simulink model "DrivetrainHevMm"  (R2020a)
settings: Solver=VariableStepAuto  StartTime=0.0  StopTime=inf  RelTol=1e-3  EnableMultiTasking=on
model workspace (MAT data in the model file):
  DiffRatio = 3.421
  EngDriveRatio = 0.813008130081
  Jengine = 0.22
  MotGbRatio = 2.45
  NF = Simulink.Parameter
  NF.Value = 2
  NF.DataType = 'auto'
  NF.Dimensions = [1 1]
  NR = Simulink.Parameter
  NR.Value = 2
  NR.DataType = 'auto'
  NR.Dimensions = [1 1]
  RWheel = 0.3
  b_axle = Simulink.Parameter
  b_axle.Value = 10
  b_axle.DataType = 'auto'
  b_axle.Dimensions = [1 1]
  b_driveshaft = Simulink.Parameter
  b_driveshaft.Value = 10
  b_driveshaft.DataType = 'auto'
  b_driveshaft.Dimensions = [1 1]
  k_axle = Simulink.Parameter
  k_axle.Value = 5000
  k_axle.DataType = 'auto'
  k_axle.Dimensions = [1 1]
  k_driveshaft = Simulink.Parameter
  k_driveshaft.Value = 1000
  k_driveshaft.DataType = 'auto'
  k_driveshaft.Dimensions = [1 1]
  wc_shaft = Simulink.Parameter
  wc_shaft.Value = 1000
  wc_shaft.DataType = 'auto'
  wc_shaft.Dimensions = [1 1]
libraries: autolibpowerinfoutils x8, autolibsharedcoupling x7, autolibshareddiff x4, autolibshared x3, autolibtransamt x1
(part 1 of 3)
settings Model: ModifiedByFormat=The MathWorks, Inc.  SimulationMode=accelerator  PauseTimes=10  Creator=The MathWorks, Inc.  LastModifiedBy=The MathWorks, Inc.
settings SolverCC: DecoupledContinuousIntegration=on
settings DataIOCC: DSMLogging=off  ReturnWorkspaceOutputs=off
settings DebuggingCC: MergeDetectMultiDrivingBlocksExec=none  ArithmeticOperatorsInVariantConditions=warning
settings ModelReferenceCC: PropagateSignalLabelsOutOfModel=off
settings SFSimCC: SimUseLocalCustomCode=off  CustomCodeUndefinedFunction=UseInterfaceOnly
settings RTWCC: RTWUseLocalCustomCode=off
settings CodeAppCC: StateflowObjectComments=on
settings GRTTargetCC: TargetLangStandard=C89/C90 (ANSI)
settings ConfigComp: CovMetricSettings=dsw  CovHtmlReporting=on  CovSaveCumulativeToWorkspaceVar=on  CovSaveSingleToWorkspaceVar=on  CovShowResultsExplorer=off  CovExternalEMLEnable=off
settings SimscapeCC: SimscapeNormalizeSystem=off  SimscapeNominalValues={1, 'bar'; 1, 'cm^3/s'; 1, 'bar*kg/s'; 1, 'kJ/kg'; 1, 'kW'; }

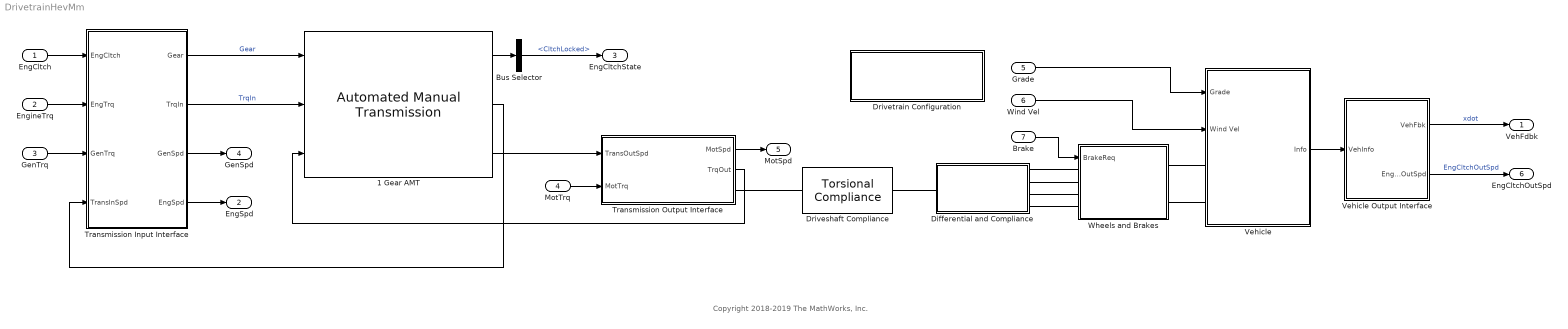
== system DrivetrainHevMm ==
  note: Copyright 2018-2019 The MathWorks, Inc.
  EngCltch : Inport  OutDataTypeStr=boolean
  EngineTrq : Inport  Port=2
  GenTrq : Inport  Port=3
  MotTrq : Inport  Port=4
  Grade : Inport  Port=5
  Wind Vel : Inport  Port=6
  Brake : Inport  Port=7
  1 Gear AMT : autolibtransamt/Automated Manual Transmission  VariantControl=0  cntrlType=Ideal integrated controller  TransEffModelPopup=Gear only  Jin=Jengine  bin=.0011  omegain_o=0  G=[0, 1]  Trq_bpts=[25, 50, 75, 100, 150, 200, 250]  omega_bpts=[52.4 78.5 105 131 157 183 209 262 314 419 524]  Temp_bpts=[313 358]  N=[EngDriveRatio EngDriveRatio]  Jout=[0.03 0.03]  bout=[.001 .001]  eta=[0.95, 0.95]  eta_tbl=reshape([0.53 0.71 0.77 0.79 0.82 0.82 0.82 0.5 0.7 0.77 0.79 0.82 0.82 0.82 0.54 0.72 0.78 0.81 0.83 0.82 0.82 0.56 0.73 0.79 0.81 0.84 0.82 0.82 0.58 0.74 0.79 0.82 0.84 0.82 0.82 0.57 0.74 0.79 0.82 0.84 0.82 0.82 0.58 0.74 0.79 0.82 0.84 0.82 0.82 0.58 0.74 0.79 0.82 0.84 0.82 0.82 0.57 0.74 0.8 0.82 0.85 0.82 0.82 0.55 0.73 0.78 0.81 0.84 0.82 0.82 0.51 0.71 0.77 0.81 0.84 0.82 0.82 0.53 0.71 0.77 0.79 0.82 0.82 0.82 0.5 0.7 0.77 0.79 0.82 0.82 0.82 0.54 0.72 0.78 0.81 0.83 0.82 0.82 0.56 0.73 0.79 0.81 0.84 0.82 0.82 0.58 0.74 0.79 0.82 0.84 0.82 0.82 0.57 0.74 0.79 0.82 0.84 0.82 0.82 0.58 0.74 0.79 0.82 0.84 0.82 0.82 0.58 0.74 0.79 0.82 0.84 0.82 0.82 0.57 0.74 0.8 0.82 0.85 0.82 0.82 0.55 0.73 0.78 0.81 0.84 0.82 0.82 0.51 0.71 0.77 0.81 0.84 0.82 0.82 0.53 0.71 0.77 0.79 0.82 0.82 0.82 0.5 0.7 0.77 0.79 0.82 0.82 0.82 0.54 0.72 0.78 0.81 0.83 0.82 0.82 0.56 0.73 0.79 0.81 0.84 0.82 0.82 0.58 0.74 0.79 0.82 0.84 0.82 0.82 0.57 0.74 0.79 0.82 0.84 0.82 0.82 0.58 0.74 0.79 0.82 0.84 0.82 0.82 0.58 0.74 0.79 0.82 0.84 0.82 0.82 0.57 0.74 0.8 0.82 0.85 0.82 0.82 0.55 0.73 0.78 0.81 0.84 0.82 0.82 0.51 0.71 0.77 0.81 0.84 0.82 0.82 0.7 0.79 0.82 0.83 0.84 0.84 0.84 0.63 0.76 0.8 0.82 0.83 0.84 0.84 0.58 0.74 0.79 0.81 0.83 0.84 0.84 0.58 0.74 0.79 0.81 0.83 0.84 0.84 0.58 0.74 0.79 0.81 0.84 0.84 0.84 0.57 0.73 0.78 0.81 0.84 0.85 0.84 0.57 0.73 0.79 0.81 0.84 0.85 0.84 0.56 0.73 0.78 0.81 0.83 0.85 0.84 0.55 0.73 0.78 0.81 0.84 0.85 0.84 0.52 0.71 0.77 0.8 0.83 0.85 0.84 0.48 0.69 0.76 0.79 0.83 0.84 0.84 0.64 0.76 0.8 0.81 0.83 0.84 0.84 0.56 0.73 0.78 0.8 0.83 0.84 0.84 0.54 0.71 0.77 0.8 0.82 0.84 0.84 0.53 0.71 0.77 0.8 0.83 0.84 0.84 0.51 0.71 0.77 0.8 0.83 0.84 0.85 0.52 0.7 0.77 0.8 0.83 0.84 0.85 0.51 0.71 0.76 0.79 0.83 0.84 0.85 0.5 0.69 0.76 0.79 0.82 0.84 0.85 0.45 0.68 0.75 0.78 0.82 0.84 0.85 0.43 0.67 0.74 0.78 0.81 0.83 0.84 0.38 0.63 0.71 0.75 0.8 0.82 0.83 0.65 0.79 0.84 0.85 0.88 0.89 0.89 0.56 0.75 0.81 0.83 0.86 0.88 0.89 0.52 0.72 0.79 0.83 0.86 0.88 0.88 0.51 0.72 0.79 0.83 0.86 0.88 0.89 0.49 0.71 0.78 0.82 0.86 0.88 0.89 0.47 0.7 0.78 0.82 0.86 0.87 0.88 0.45 0.69 0.77 0.81 0.85 0.87 0.88 0.4 0.67 0.75 0.8 0.84 0.86 0.88 0.3 0.64 0.73 0.78 0.83 0.86 0.87 0.17 0.55 0.67 0.73 0.8 0.83 0.85 0.089 0.45 0.61 0.69 0.77 0.81 0.83 0.61 0.75 0.82 0.84 0.87 0.87 0.88 0.54 0.73 0.8 0.82 0.86 0.87 0.88 0.51 0.71 0.79 0.82 0.86 0.87 0.88 0.52 0.72 0.79 0.82 0.86 0.87 0.89 0.52 0.72 0.8 0.83 0.86 0.88 0.89 0.53 0.72 0.79 0.82 0.86 0.87 0.89 0.5 0.7 0.78 0.82 0.86 0.88 0.88 0.46 0.69 0.77 0.81 0.85 0.87 0.88 0.4 0.67 0.75 0.8 0.83 0.86 0.88 0.33 0.64 0.73 0.78 0.83 0.85 0.87 0.33 0.64 0.73 0.78 0.83 0.85 0.87 0.78 0.85 0.87 0.88 0.89 0.89 0.89 0.73 0.83 0.86 0.88 0.89 0.89 0.89 0.72 0.83 0.86 0.88 0.89 0.89 0.89 0.72 0.83 0.87 0.89 0.9 0.89 0.89 0.72 0.83 0.87 0.88 0.9 0.89 0.89 0.71 0.83 0.87 0.88 0.9 0.89 0.89 0.71 0.83 0.86 0.88 0.9 0.89 0.89 0.7 0.82 0.86 0.88 0.9 0.89 0.89 0.69 0.82 0.86 0.88 0.9 0.89 0.89 0.67 0.81 0.86 0.88 0.9 0.89 0.89 0.63 0.79 0.85 0.87 0.89 0.89 0.89 0.78 0.85 0.87 0.88 0.89 0.89 0.89 0.73 0.83 0.86 0.88 0.89 0.89 0.89 0.72 0.83 0.86 0.88 0.89 0.89 0.89 0.72 0.83 0.87 0.89 0.9 0.89 0.89 0.72 0.83 0.87 0.88 0.9 0.89 0.89 0.71 0.83 0.87 0.88 0.9 0.89 0.89 0.71 0.83 0.86 0.88 0.9 0.89 0.89 0.7 0.82 0.86 0.88 0.9 0.89 0.89 0.69 0.82 0.86 0.88 0.9 0.89 0.89 0.67 0.81 0.86 0.88 0.9 0.89 0.89 0.63 0.79 0.85 0.87 0.89 0.89 0.89 0.78 0.85 0.87 0.88 0.89 0.89 0.89 0.73 0.83 0.86 0.88 0.89 0.89 0.89 0.72 0.83 0.86 0.88 0.89 0.89 0.89 0.72 0.83 0.87 0.89 0.9 0.89 0.89 0.72 0.83 0.87 0.88 0.9 0.89 0.89 0.71 0.83 0.87 0.88 0.9 0.89 0.89 0.71 0.83 0.86 0.88 0.9 0.89 0.89 0.7 0.82 0.86 0.88 0.9 0.89 0.89 0.69 0.82 0.86 0.88 0.9 0.89 0.89 0.67 0.81 0.86 0.88 0.9 0.89 0.89 0.63 0.79 0.85 0.87 0.89 0.89 0.89 0.82 0.87 0.88 0.89 0.89 0.89 0.89 0.81 0.87 0.89 0.89 0.9 0.9 0.89 0.76 0.85 0.87 0.89 0.9 0.89 0.89 0.72 0.83 0.86 0.88 0.89 0.89 0.89 0.72 0.83 0.86 0.88 0.89 0.9 0.89 0.71 0.82 0.86 0.88 0.89 0.9 ...(+1314 chars))  omegaout_o=0  G_o=0  tauc=.02  ts=0.02  tc=.5  R=.2  K_c=5e3  mus=0.35  muk=0.3  ClutchLocked=off  SynchLocked=off  maxAbsSpd=5e3
      settings: SourceProductBaseCode=PW
  Bus Selector : BusSelector  OutputSignals=Cltch.CltchLocked
  Differential and Compliance : Subsystem  Variant=on  VariantControlMode=Label  LabelModeActiveChoice=0
  Driveshaft Compliance : autolibsharedcoupling/Torsional Compliance  port_config=Two-way connection  extInfo=off  k=k_driveshaft  b=b_driveshaft  theta_o=0  domega_o=0  omega_c=wc_shaft  blkID=0  aMode=1
      settings: SourceProductBaseCode=PW,MT,VE,VP
  Drivetrain Configuration : Subsystem  mask(Drivetrain Configuration){drivetrainMode=Front Wheel Drive}
      mask prompts: drivetrainMode "Drivetrain Mode"
      mask help: Use this block to configure the dirvetrain mode.
      settings: AttributesFormatString=Active Mode: %<drivetrainMode>
      mask TypeOptions drivetrainMode: Front Wheel Drive | Rear Wheel Drive | All Wheel Drive
      mask Callback drivetrainMode:
      | switch get_param(gcb,'drivetrainMode')
      |     case 'Front Wheel Drive'
      |         set_param([bdroot '/Differential and Compliance'],'OverrideUsingVariant','0')
      |     case 'Rear Wheel Drive'
      |         set_param([bdroot '/Differential and Compliance'],'OverrideUsingVariant','1')
      |     case 'All Wheel Drive'
      |         set_param([bdroot '/Differential and Compliance'],'OverrideUsingVariant','2')
      |     otherwise
      |         set_param([bdroot '/Differential and Compliance'],'OverrideUsingVariant','0')
      | end
      mask Display: disp('Double click to configure drivetrain')
  Transmission Input Interface : Subsystem
  Transmission Output Interface : Subsystem
  Vehicle : Subsystem
  Vehicle Output Interface : Subsystem
  Wheels and Brakes : Subsystem  VariantControl=0
  VehFdbk : Outport  VectorParamsAs1DForOutWhenUnconnected=off
  EngSpd : Outport  Port=2  VectorParamsAs1DForOutWhenUnconnected=off  BusOutputAsStruct=on
  EngCltchState : Outport  Port=3  VectorParamsAs1DForOutWhenUnconnected=off  BusOutputAsStruct=on
  GenSpd : Outport  Port=4  VectorParamsAs1DForOutWhenUnconnected=off  BusOutputAsStruct=on
  MotSpd : Outport  Port=5  VectorParamsAs1DForOutWhenUnconnected=off  BusOutputAsStruct=on
  EngCltchOutSpd : Outport  Port=6  VectorParamsAs1DForOutWhenUnconnected=off  BusOutputAsStruct=on
  wires:
  Brake/1 -> Wheels and Brakes/1(BrakeReq)
  1 Gear AMT/2 -> Transmission Input Interface/4(TransInSpd)
  1 Gear AMT/1 -> Bus Selector/1
  Bus Selector/1 -> EngCltchState/1  "<CltchLocked>"
  Transmission Input Interface/1(Gear) -> 1 Gear AMT/1  "Gear"
  Transmission Input Interface/2(TrqIn) -> 1 Gear AMT/2  "TrqIn"
  EngCltch/1 -> Transmission Input Interface/1(EngCltch)
  EngineTrq/1 -> Transmission Input Interface/2(EngTrq)
  GenTrq/1 -> Transmission Input Interface/3(GenTrq)
  Vehicle/1(Info) -> Vehicle Output Interface/1(VehInfo)
  Vehicle Output Interface/1(VehFbk) -> VehFdbk/1  "xdot"
  Vehicle Output Interface/2(EngCltchOutSpd) -> EngCltchOutSpd/1  "EngCltchOutSpd"
  Grade/1 -> Vehicle/1(Grade)
  Wind Vel/1 -> Vehicle/2(Wind Vel)
  1 Gear AMT/3 -> Transmission Output Interface/1(TransOutSpd)
  MotTrq/1 -> Transmission Output Interface/2(MotTrq)
  Transmission Output Interface/1(MotSpd) -> MotSpd/1
  Transmission Output Interface/2(TrqOut) -> 1 Gear AMT/3
  Transmission Input Interface/3(GenSpd) -> GenSpd/1
  Transmission Input Interface/4(EngSpd) -> EngSpd/1
  connections:
  Differential and Compliance/LConn1 -- Driveshaft Compliance/RConn1
  Wheels and Brakes/RConn1 -- Vehicle/LConn1
  Differential and Compliance/RConn1 -- Wheels and Brakes/LConn1
  Differential and Compliance/RConn3 -- Wheels and Brakes/LConn3
  Differential and Compliance/RConn2 -- Wheels and Brakes/LConn2
  Differential and Compliance/RConn4 -- Wheels and Brakes/LConn4
  Vehicle/LConn2 -- Wheels and Brakes/RConn2
  Driveshaft Compliance/LConn1 -- Transmission Output Interface/RConn1

== system DrivetrainHevMm/Differential and Compliance ==
  All Wheel Drive : Subsystem  VariantControl=2
  Front Wheel Drive : Subsystem  VariantControl=0
  Rear Wheel Drive : Subsystem  VariantControl=1
  D : PMIOPort  Side=Left
  FA1 : PMIOPort  Port=2  Side=Right
  FA2 : PMIOPort  Port=3  Side=Right
  RA1 : PMIOPort  Port=4  Side=Right
  RA2 : PMIOPort  Port=5  Side=Right

== system DrivetrainHevMm/Drivetrain Configuration ==

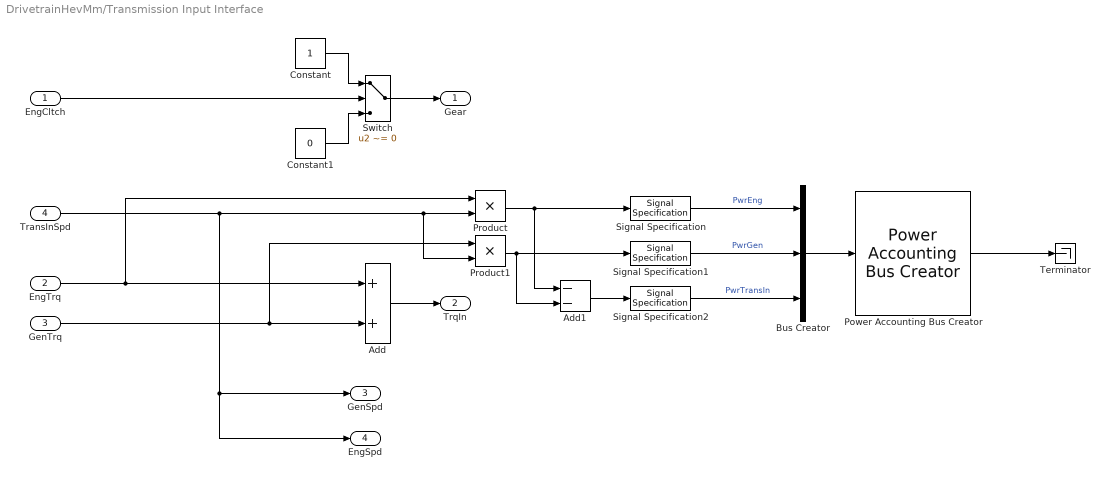
== system DrivetrainHevMm/Transmission Input Interface ==
  EngCltch : Inport  OutDataTypeStr=boolean
  EngTrq : Inport  Port=2
  GenTrq : Inport  Port=3
  TransInSpd : Inport  Port=4
  Add : Sum
  Add1 : Sum  Inputs=--
  Bus Creator : BusCreator  Inputs=3
  Constant : Constant
  Constant1 : Constant  Value=0
  Power Accounting Bus Creator : autolibpowerinfoutils/Power Accounting Bus Creator  AssctBlkSelPopup=Parent  RefBlkName='libraryname/blkname'  PwrTrnsfrdCheckBox=on  PwrNotTrnsfrdCheckBox=off  PwrStoredCheckBox=off  aMode=aMode
      settings: SourceProductBaseCode=PW,MT,VE,VP
  Product : Product
  Product1 : Product
  Signal Specification : SignalSpecification  Unit=W
  Signal Specification1 : SignalSpecification  Unit=W
  Signal Specification2 : SignalSpecification  Unit=W
  Switch : Switch  Criteria=u2 ~= 0
  Terminator : Terminator
  Gear : Outport  VectorParamsAs1DForOutWhenUnconnected=off
  TrqIn : Outport  Port=2  VectorParamsAs1DForOutWhenUnconnected=off
  GenSpd : Outport  Port=3  VectorParamsAs1DForOutWhenUnconnected=off
  EngSpd : Outport  Port=4  VectorParamsAs1DForOutWhenUnconnected=off
  wires:
  GenTrq/1 -> Product1/1, Add/2
  Add/1 -> TrqIn/1
  EngCltch/1 -> Switch/2
  EngTrq/1 -> Product/1, Add/1
  Constant/1 -> Switch/1
  Constant1/1 -> Switch/3
  Switch/1 -> Gear/1
  Bus Creator/1 -> Power Accounting Bus Creator/1
  Product/1 -> Add1/1, Signal Specification/1
  Signal Specification/1 -> Bus Creator/1  "PwrEng"
  TransInSpd/1 -> GenSpd/1, EngSpd/1, Product1/2, Product/2
  Product1/1 -> Add1/2, Signal Specification1/1
  Signal Specification1/1 -> Bus Creator/2  "PwrGen"
  Add1/1 -> Signal Specification2/1
  Signal Specification2/1 -> Bus Creator/3  "PwrTransIn"
  Power Accounting Bus Creator/1 -> Terminator/1

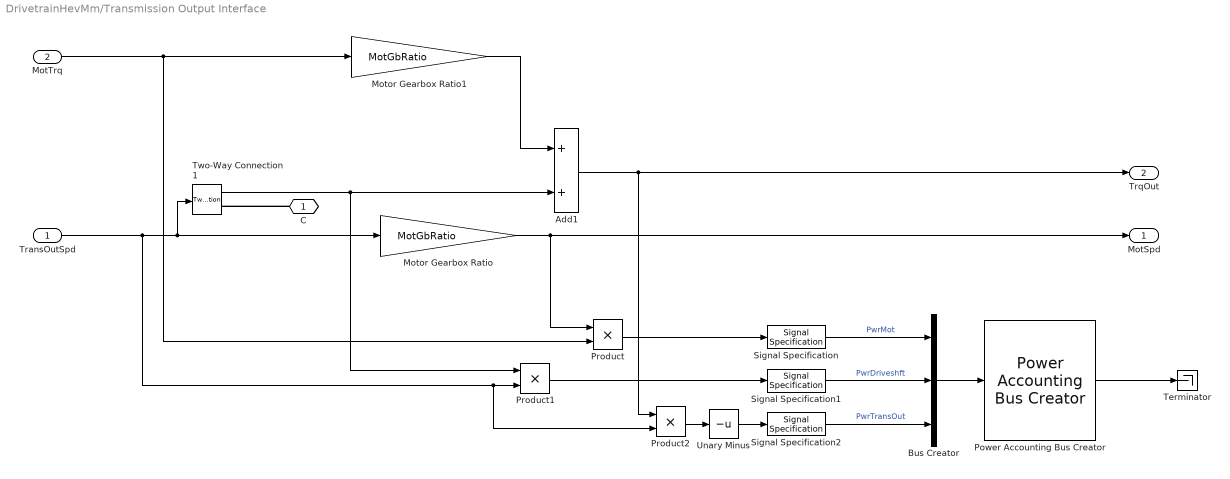
== system DrivetrainHevMm/Transmission Output Interface ==
  TransOutSpd : Inport
  MotTrq : Inport  Port=2
  Add1 : Sum
  Bus Creator : BusCreator  Inputs=3
  Motor Gearbox Ratio : Gain  Gain=MotGbRatio
  Motor Gearbox Ratio1 : Gain  Gain=MotGbRatio
  Power Accounting Bus Creator : autolibpowerinfoutils/Power Accounting Bus Creator  AssctBlkSelPopup=Parent  RefBlkName='libraryname/blkname'  PwrTrnsfrdCheckBox=on  PwrNotTrnsfrdCheckBox=off  PwrStoredCheckBox=off  aMode=aMode
      settings: SourceProductBaseCode=PW,MT,VE,VP
  Product : Product
  Product1 : Product
  Product2 : Product
  Signal Specification : SignalSpecification  Unit=W
  Signal Specification1 : SignalSpecification  Unit=W
  Signal Specification2 : SignalSpecification  Unit=W
  Terminator : Terminator
  Two-Way Connection1 : TwoWayConnection
  Unary Minus : UnaryMinus
  C : PMIOPort  Side=Right
  MotSpd : Outport  VectorParamsAs1DForOutWhenUnconnected=off
  TrqOut : Outport  Port=2  VectorParamsAs1DForOutWhenUnconnected=off
  wires:
  Add1/1 -> TrqOut/1, Product2/1
  Motor Gearbox Ratio/1 -> MotSpd/1, Product/1
  Motor Gearbox Ratio1/1 -> Add1/1
  Bus Creator/1 -> Power Accounting Bus Creator/1
  Power Accounting Bus Creator/1 -> Terminator/1
  Signal Specification2/1 -> Bus Creator/3  "PwrTransOut"
  Signal Specification1/1 -> Bus Creator/2  "PwrDriveshft"
  MotTrq/1 -> Product/2, Motor Gearbox Ratio1/1
  TransOutSpd/1 -> Product2/2, Product1/2, Two-Way Connection1/1, Motor Gearbox Ratio/1
  Product/1 -> Signal Specification/1
  Two-Way Connection1/1 -> Product1/1, Add1/2
  Product1/1 -> Signal Specification1/1
  Signal Specification/1 -> Bus Creator/1  "PwrMot"
  Product2/1 -> Unary Minus/1
  Unary Minus/1 -> Signal Specification2/1
  connections:
  C/RConn1 -- Two-Way Connection1/RConn1

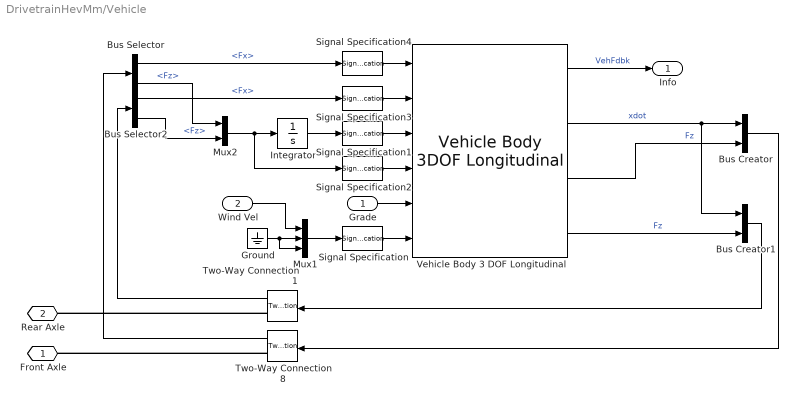
== system DrivetrainHevMm/Vehicle ==
  Grade : Inport  Unit=deg
  Wind Vel : Inport  Port=2  Unit=m/s
  Bus Creator : BusCreator  Inputs=2
  Bus Creator1 : BusCreator  Inputs=2
  Bus Selector : BusSelector  OutputSignals=Fx,Fz
  Bus Selector2 : BusSelector  OutputSignals=Fx,Fz
  Ground : Ground
  Integrator : Integrator
  Mux1 : Mux  Inputs=3
  Mux2 : Mux  Inputs=2
  Signal Specification : SignalSpecification  Unit=m/s
  Signal Specification1 : SignalSpecification  Unit=m
  Signal Specification2 : SignalSpecification  Unit=m/s
  Signal Specification3 : SignalSpecification  Unit=N
  Signal Specification4 : SignalSpecification  Unit=N
  Two-Way Connection1 : TwoWayConnection
  Two-Way Connection8 : TwoWayConnection
  Vehicle Body 3 DOF Longitudinal : autolibshared/Vehicle Body 3DOF Longitudinal  VariantControl=SL  groundType=Axle displacement, velocity  aMode=1  extFMode=off  extMMode=off  extTamb=off  NF=NF  NR=NR  m=1.7232e+03  a=1.56  b=1.22  h=.5  Cd=.29  Af=2.27  x_o=0  xdot_o=0  Cl=.1  z_o=-.35  zdot_o=0  Iyy=3000  Cpm=.1  theta_o=0  q_o=0  FskF=[-50, -1, 0, 2, 3, 52].*1.25e4  dzsF=[-5e-3, -1e-4, 0, .2, .2001, .2051]  FsbF=[-10000 -100 -10 0 10 100 10000]  dzdotsF=[-10 -1 -.1 0 .1 1 10]  FskR=[-50, -1, 0, 2, 3, 52].*7.5e3  dzsR=[-5e-3, -1e-4, 0, .2, .2001, .2051]  FsbR=[-10000 -100 -10 0 10 100 10000]  dzdotsR=[-10 -1 -.1 0 .1 1 10]  Pabs=101325  T=273  g=9.81  blkID=0
      settings: SourceProductBaseCode=PW,MT,VE,VP
  Front Axle : PMIOPort  Side=Left
  Rear Axle : PMIOPort  Port=2  Side=Left
  Info : Outport  VectorParamsAs1DForOutWhenUnconnected=off
  wires:
  Two-Way Connection1/1 -> Bus Selector2/1
  Bus Selector2/2 -> Mux2/2  "<Fz>"
  Bus Selector2/1 -> Signal Specification3/1  "<Fx>"
  Bus Selector/2 -> Mux2/1  "<Fz>"
  Bus Selector/1 -> Signal Specification4/1  "<Fx>"
  Bus Creator1/1 -> Two-Way Connection1/1
  Bus Creator/1 -> Two-Way Connection8/1
  Signal Specification4/1 -> Vehicle Body 3 DOF Longitudinal/1
  Signal Specification3/1 -> Vehicle Body 3 DOF Longitudinal/2
  Signal Specification2/1 -> Vehicle Body 3 DOF Longitudinal/4
  Signal Specification1/1 -> Vehicle Body 3 DOF Longitudinal/3
  Signal Specification/1 -> Vehicle Body 3 DOF Longitudinal/6
  Grade/1 -> Vehicle Body 3 DOF Longitudinal/5
  Wind Vel/1 -> Mux1/1
  Integrator/1 -> Signal Specification1/1
  Mux2/1 -> Signal Specification2/1, Integrator/1
  Vehicle Body 3 DOF Longitudinal/4 -> Bus Creator1/2  "Fz"
  Mux1/1 -> Signal Specification/1
  Ground/1 -> Mux1/3, Mux1/2
  Vehicle Body 3 DOF Longitudinal/1 -> Info/1  "VehFdbk"
  Two-Way Connection8/1 -> Bus Selector/1
  Vehicle Body 3 DOF Longitudinal/2 -> Bus Creator/1, Bus Creator1/1  "xdot"
  Vehicle Body 3 DOF Longitudinal/3 -> Bus Creator/2  "Fz"
  connections:
  Two-Way Connection1/RConn1 -- Rear Axle/RConn1
  Two-Way Connection8/RConn1 -- Front Axle/RConn1

== system DrivetrainHevMm/Vehicle Output Interface ==
  VehInfo : Inport
  1/wheel radius : Gain  Gain=1/RWheel
  Bus Selector1 : BusSelector  OutputSignals=BdyFrm.Cg.Vel.xdot
  Gain : Gain  Gain=EngDriveRatio
  Motor Gearbox Ratio2 : Gain  Gain=DiffRatio
  VehFbk : Outport  VectorParamsAs1DForOutWhenUnconnected=off
  EngCltchOutSpd : Outport  Port=2  VectorParamsAs1DForOutWhenUnconnected=off
  wires:
  Bus Selector1/1 -> VehFbk/1, 1/wheel radius/1  "<xdot>"
  Gain/1 -> EngCltchOutSpd/1
  VehInfo/1 -> Bus Selector1/1
  Motor Gearbox Ratio2/1 -> Gain/1
  1/wheel radius/1 -> Motor Gearbox Ratio2/1
